simulink model "system_simulink"  (R2015b)
settings: Solver=VariableStepAuto  StartTime=0.0  StopTime=10.0  RelTol=1e-3
settings Model: Creator=一宁宝宝  LastModifiedBy=一宁宝宝

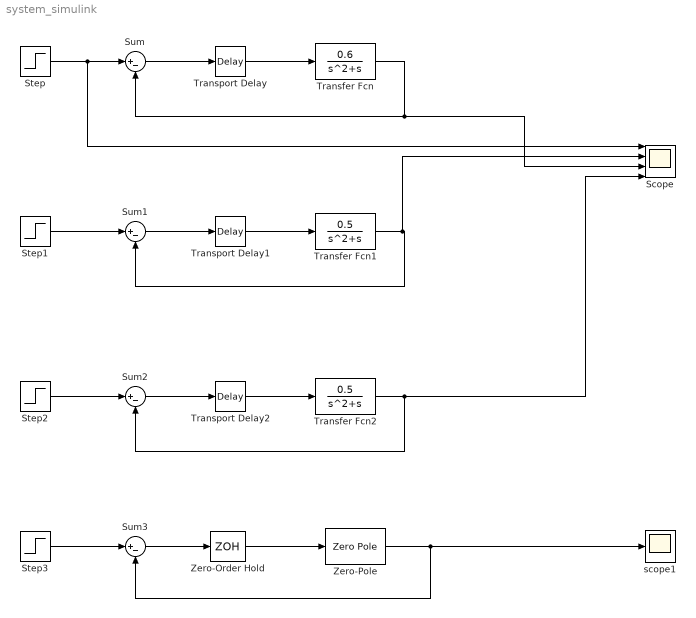
== system system_simulink ==
  Scope : Scope  NumInputPorts=4
  Step{,1..3} (4 alike) : Step  SampleTime=0
  Sum{,1..3} (4 alike) : Sum  Inputs=|+-
  Transfer Fcn : TransferFcn  Numerator=[0.6]  Denominator=[1 1 0]
  Transfer Fcn1 : TransferFcn  Numerator=[0.5]  Denominator=[1 1 0]
  Transfer Fcn2 : TransferFcn  Numerator=[0.5]  Denominator=[1 1 0]
  Transport Delay : TransportDelay  DelayTime=0.5
  Transport Delay1 : TransportDelay  DelayTime=0.5
  Transport Delay2 : TransportDelay  DelayTime=0.3
  Zero-Order Hold : ZeroOrderHold  SampleTime=0.01
  Zero-Pole : ZeroPole  Zeros=[]  Poles=[0 -1]
  scope1 : Scope
  wires:
  Step/1 -> Scope/1, Sum/1
  Sum/1 -> Transport Delay/1
  Transport Delay/1 -> Transfer Fcn/1
  Transfer Fcn/1 -> Scope/3, Sum/2
  Step1/1 -> Sum1/1
  Sum1/1 -> Transport Delay1/1
  Transport Delay1/1 -> Transfer Fcn1/1
  Transfer Fcn1/1 -> Scope/2, Sum1/2
  Step2/1 -> Sum2/1
  Sum2/1 -> Transport Delay2/1
  Transport Delay2/1 -> Transfer Fcn2/1
  Transfer Fcn2/1 -> Scope/4, Sum2/2
  Step3/1 -> Sum3/1
  Sum3/1 -> Zero-Order Hold/1
  Zero-Order Hold/1 -> Zero-Pole/1
  Zero-Pole/1 -> scope1/1, Sum3/2
